simulink model "gm_sampleModel1614_4_sub"  (R2023a)
settings: Solver=VariableStepAuto  StartTime=0.0  StopTime=10.0  RelTol=1e-3
libraries: hdlsllib x1
settings Model: Creator=user1  LastModifiedBy=user1
settings OptimizationCC: BlockReduction=off  ConditionallyExecuteInputs=off
settings DebuggingCC: InheritedTsInSrcMsg=none

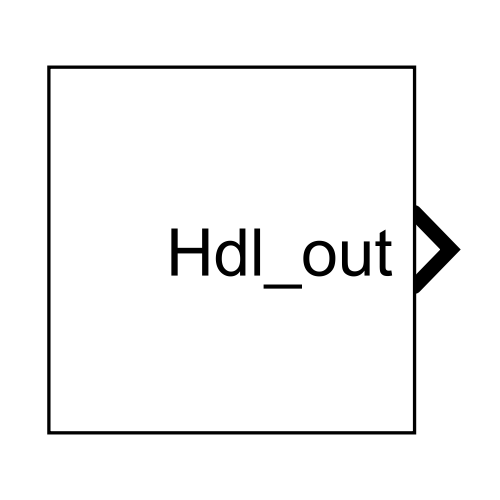
[thumbnail: Simulink's stored preview of the top-level diagram]
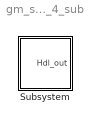
== system gm_sampleModel1614_4_sub ==
  Subsystem : Subsystem

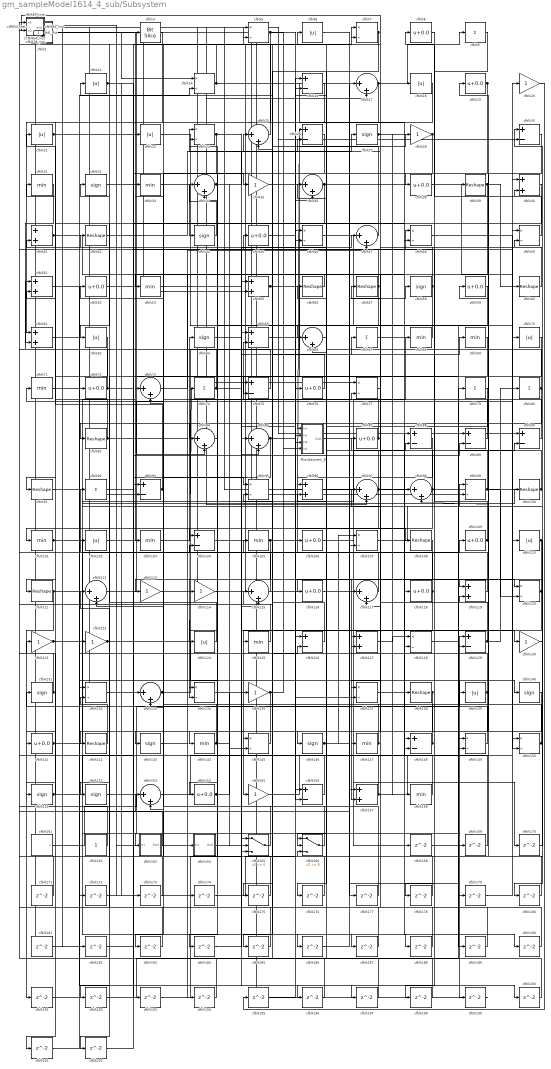
== system gm_sampleModel1614_4_sub/Subsystem ==
  Mysubsystem_8 : Subsystem
  cfblk1 : Subsystem  mask(Detect Rise Nonnegative){vinit=double(0), InputProcessing=Elements as channels (sample based), OutDataTypeStr=uint8}
      mask prompts: vinit "Simulink:masks:InitialCondition_MP"; InputProcessing "Simulink:masks:InputProcessing_MP"; OutDataTypeStr "Simulink:masks:OutputDataType_MP"
      mask help: Simulink:masks:DetectRiseNonnegative_MD
      mask init:
      | InputProcessing = 'Elements as channels (sample based)';
      | OutDataTypeStr = 'uint8';
      | vinit = double(0);
      mask TypeOptions InputProcessing: Simulink:masks:ColumnsAsChannelsFrameBased | Simulink:masks:ElementsAsChannelsSampleBased
      mask TypeOptions OutDataTypeStr: Simulink:masks:uint8 | Simulink:masks:boolean
      mask Display: fprintf('U >= 0\n&  NOT\nU/z >= 0')
  cfblk{39,42,56..57,60,82,91,100,108,111,138,142} (12 alike) : Reshape
  cfblk{31,33,53,68..69,71,101,103,105,125,144,147,158} (13 alike) : MinMax  OutDataTypeStr=uint8
  cfblk{6,12,18,21,23,62,70,102,110,124,139} (11 alike) : Abs  OutDataTypeStr=uint8  SaturateOnIntegerOverflow=off
  cfblk{16,26,30,75,88..90,93,104,126,129,148,156} (13 alike) : Sum  Inputs=+-  OutDataTypeStr=uint8
  cfblk{8,19,38,45,52,59,72,76,87,106,109,116,118,141,154} (15 alike) : Bias  Bias=0.0  SaturateOnIntegerOverflow=off
  cfblk{5,7,14,24,46,48,50,77,95,99,107,120,128,132,134,137,145,149..150} (19 alike) : Product  Inputs=*/  OutDataTypeStr=uint8  RndMeth=Zero  SaturateOnIntegerOverflow=on
  cfblk{17,25,34,36,47,66,73,84..85,97..98,112,115,117,133,153} (16 alike) : Sum  Inputs=|++  OutDataTypeStr=uint8
  cfblk{20,28,35,113..114,121..122,130,135,155} (10 alike) : Gain  OutDataTypeStr=uint8
  cfblk{40..41,51,55,61,65,96,119,127,157} (10 alike) : Sum  OutDataTypeStr=uint8
  cfblk11_inst : Subsystem
  cfblk123_inst : Subsystem
  cfblk{27,32,44,58,64,131,140,143,146,151..152} (11 alike) : Signum
  cfblk136_inst : Subsystem
  cfblk13_inst : Subsystem
  cfblk15_inst : Subsystem
  cfblk161 : Subsystem  mask(Counter Free-Running){NumBits=double(16), tsamp=double(-1)}
      mask prompts: NumBits "Simulink:masks:NumberOfBits_MP"; tsamp "Simulink:masks:SampleTime_MP"
      mask help: Simulink:masks:CounterFreeRunning_MD
  cfblk162 : Constant  OutDataTypeStr=uint8  SampleTime=-1
  cfblk163 : Subsystem
  cfblk164 : Subsystem
  cfblk165 : Switch  OutDataTypeStr=uint8  SaturateOnIntegerOverflow=off  InputSameDT=off
  cfblk166 : Switch  OutDataTypeStr=uint8  SaturateOnIntegerOverflow=off  InputSameDT=off
  cfblk{168..202} (35 alike) : Delay  SampleTime=1
  cfblk2 : Constant  Value=0  OutDataTypeStr=uint8  SampleTime=1
  cfblk22_inst : Subsystem
  cfblk29_inst : Subsystem
  cfblk3 : hdlsllib/Logic and Bit Operations/Bit Slice  lidx=7  ridx=0
  cfblk37_inst : Subsystem
  cfblk43_inst : Subsystem
  cfblk49_inst : Subsystem
  cfblk4_inst : Subsystem
  cfblk54_inst : Subsystem
  cfblk{9,67,74,79..80,92} (6 alike) : Sum  Inputs=+  OutDataTypeStr=uint8
  cfblk78_inst : Subsystem
  cfblk83_inst : Subsystem
  cfblk94_inst : Subsystem
  Hdl_out : Outport  OutDataTypeStr=uint8  SampleTime=1
  wires:
  Mysubsystem_8/1(Out1) -> cfblk168/1
  cfblk1/1(Y) -> cfblk84/2, cfblk14/1
  cfblk100/1 -> cfblk43_inst/2(in2), Hdl_out/1
  cfblk101/1 -> cfblk100/1, cfblk188/1
  cfblk102/1 -> cfblk3/1
  cfblk103/1 -> cfblk64/1
  cfblk104/1 -> cfblk6/1
  cfblk105/1 -> cfblk26/1, cfblk134/2
  cfblk106/1 -> cfblk120/1
  cfblk107/1 -> cfblk50/2
  cfblk108/1 -> cfblk153/2
  cfblk109/1 -> cfblk98/2, cfblk45/1
  cfblk11_inst/1(out1) -> cfblk17/2, cfblk133/1
  cfblk110/1 -> cfblk166/3, cfblk157/2, cfblk180/1
  cfblk111/1 -> cfblk73/1, cfblk109/1, cfblk191/1, cfblk187/1
  cfblk112/1 -> cfblk40/1
  cfblk113/1 -> cfblk28/1
  cfblk114/1 -> cfblk48/1
  cfblk115/1 -> cfblk123_inst/1(in1)
  cfblk116/1 -> cfblk170/1
  cfblk117/1 -> cfblk92/1
  cfblk118/1 -> cfblk25/2, cfblk127/2
  cfblk119/1 -> cfblk15_inst/1(in1)
  cfblk12/1 -> cfblk93/1, cfblk173/1
  cfblk120/1 -> cfblk155/1, cfblk113/1, cfblk125/1
  cfblk121/1 -> cfblk88/2, cfblk99/1
  cfblk122/1 -> cfblk199/1, cfblk74/1
  cfblk123_inst/1(out1) -> cfblk98/1, cfblk164/1(In1)
  cfblk124/1 -> cfblk49_inst/1(in1)
  cfblk125/1 -> cfblk136_inst/1(in1)
  cfblk126/1 -> cfblk5/1
  cfblk127/1 -> cfblk128/1
  cfblk128/1 -> cfblk79/1
  cfblk129/1 -> cfblk15_inst/2(in2), cfblk80/1
  cfblk13_inst/1(out1) -> cfblk99/2, cfblk77/1
  cfblk130/1 -> cfblk40/2
  cfblk131/1 -> cfblk54_inst/2(in2), cfblk201/1
  cfblk132/1 -> cfblk126/2
  cfblk133/1 -> cfblk65/2, cfblk200/1
  cfblk134/1 -> cfblk55/1
  cfblk135/1 -> cfblk183/1, Mysubsystem_8/4(In4)
  cfblk136_inst/1(out1) -> cfblk182/1, cfblk181/1
  cfblk137/1 -> cfblk88/1
  cfblk138/1 -> cfblk192/1, cfblk185/1, cfblk144/1
  cfblk139/1 -> cfblk19/1, cfblk202/1, cfblk105/1
  cfblk14/1 -> cfblk94_inst/1(in1), cfblk148/1
  cfblk140/1 -> cfblk146/1
  cfblk141/1 -> cfblk46/2, cfblk163/1(In1), cfblk68/1
  cfblk142/1 -> cfblk132/2
  cfblk143/1 -> cfblk186/1
  cfblk144/1 -> cfblk52/1, cfblk165/2, cfblk71/1
  cfblk145/1 -> cfblk142/1
  cfblk146/1 -> cfblk177/1, cfblk107/1
  cfblk147/1 -> cfblk29_inst/1(in1), cfblk24/1
  cfblk148/1 -> cfblk66/2, cfblk36/1
  cfblk149/1 -> cfblk131/1
  cfblk15_inst/1(out1) -> cfblk97/2
  cfblk150/1 -> cfblk59/1, cfblk7/1
  cfblk151/1 -> cfblk121/1, cfblk103/1
  cfblk152/1 -> cfblk169/1
  cfblk153/1 -> cfblk89/1
  cfblk154/1 -> cfblk104/2, cfblk135/1
  cfblk155/1 -> cfblk138/1
  cfblk156/1 -> cfblk115/1
  cfblk157/1 -> cfblk87/1, cfblk106/1, cfblk20/1
  cfblk158/1 -> cfblk65/1
  cfblk16/1 -> cfblk141/1
  cfblk161/1(y) -> cfblk129/1
  cfblk162/1 -> cfblk4_inst/1(in1)
  cfblk163/1(Out1) -> cfblk13_inst/2(in2)
  cfblk164/1(Out1) -> cfblk67/1
  cfblk165/1 -> cfblk112/2
  cfblk166/1 -> cfblk22_inst/2(in2)
  cfblk168/1 -> cfblk90/2
  cfblk169/1 -> cfblk123_inst/2(in2)
  cfblk17/1 -> cfblk75/2, cfblk9/1
  cfblk170/1 -> cfblk30/1
  cfblk171/1 -> cfblk94_inst/2(in2)
  cfblk172/1 -> cfblk89/2
  cfblk173/1 -> cfblk29_inst/2(in2)
  cfblk174/1 -> cfblk16/2
  cfblk175/1 -> cfblk153/1
  cfblk176/1 -> cfblk34/2
  cfblk177/1 -> cfblk5/2
  cfblk178/1 -> cfblk97/1
  cfblk179/1 -> cfblk150/1
  cfblk18/1 -> cfblk175/1
  cfblk180/1 -> cfblk119/2
  cfblk181/1 -> cfblk126/1
  cfblk182/1 -> cfblk7/2
  cfblk183/1 -> cfblk49_inst/2(in2)
  cfblk184/1 -> cfblk77/2
  cfblk185/1 -> cfblk132/1
  cfblk186/1 -> cfblk17/1
  cfblk187/1 -> cfblk112/1
  cfblk188/1 -> cfblk117/2
  cfblk189/1 -> cfblk13_inst/1(in1)
  cfblk19/1 -> cfblk75/1, Mysubsystem_8/1(In1)
  cfblk190/1 -> cfblk165/1
  cfblk191/1 -> cfblk157/1
  cfblk192/1 -> cfblk149/2
  cfblk193/1 -> cfblk115/2
  cfblk194/1 -> cfblk11_inst/2(in2)
  cfblk195/1 -> cfblk156/1
  cfblk196/1 -> cfblk54_inst/1(in1)
  cfblk197/1 -> cfblk37_inst/2(in2)
  cfblk198/1 -> cfblk95/2
  cfblk199/1 -> cfblk1/1(U)
  cfblk2/1 -> cfblk174/1
  cfblk20/1 -> cfblk195/1
  cfblk200/1 -> cfblk96/2
  cfblk201/1 -> cfblk14/2
  cfblk202/1 -> cfblk23/1
  cfblk21/1 -> cfblk48/2, cfblk35/1
  cfblk22_inst/1(out1) -> cfblk18/1
  cfblk23/1 -> cfblk139/1
  cfblk24/1 -> cfblk85/1, cfblk133/2
  cfblk25/1 -> cfblk43_inst/1(in1)
  cfblk26/1 -> cfblk156/2
  cfblk27/1 -> cfblk190/1, cfblk158/1
  cfblk28/1 -> cfblk154/1, cfblk184/1
  cfblk29_inst/1(out1) -> cfblk117/1
  cfblk3/1 -> cfblk61/1
  cfblk30/1 -> cfblk149/1
  cfblk31/1 -> cfblk61/2
  cfblk32/1 -> cfblk118/1
  cfblk33/1 -> cfblk44/1
  cfblk34/1 -> cfblk26/2, cfblk145/2, Mysubsystem_8/2(In2)
  cfblk35/1 -> cfblk119/1
  cfblk36/1 -> cfblk62/1, cfblk104/1
  cfblk37_inst/1(out1) -> cfblk30/2
  cfblk38/1 -> cfblk150/2
  cfblk39/1 -> cfblk73/2, cfblk60/1, cfblk127/1
  cfblk4_inst/1(out1) -> cfblk72/1, cfblk122/1
  cfblk40/1 -> cfblk111/1
  cfblk41/1 -> cfblk194/1, cfblk193/1, cfblk128/2
  cfblk42/1 -> cfblk27/1
  cfblk43_inst/1(out1) -> cfblk171/1
  cfblk44/1 -> cfblk34/1
  cfblk45/1 -> cfblk76/1
  cfblk46/1 -> cfblk110/1
  cfblk47/1 -> cfblk12/1
  cfblk48/1 -> cfblk70/1
  cfblk49_inst/1(out1) -> cfblk37_inst/1(in1)
  cfblk5/1 -> cfblk91/1, cfblk36/2, cfblk137/2
  cfblk50/1 -> cfblk8/1
  cfblk51/1 -> cfblk197/1
  cfblk52/1 -> cfblk85/2
  cfblk53/1 -> cfblk46/1
  cfblk54_inst/1(out1) -> cfblk39/1
  cfblk55/1 -> cfblk47/1, cfblk148/2
  cfblk56/1 -> cfblk53/1
  cfblk57/1 -> cfblk83_inst/1(in1), cfblk124/1
  cfblk58/1 -> cfblk24/2, cfblk137/1, Mysubsystem_8/3(In3)
  cfblk59/1 -> cfblk166/2
  cfblk6/1 -> cfblk179/1
  cfblk60/1 -> cfblk11_inst/1(in1)
  cfblk61/1 -> cfblk172/1
  cfblk62/1 -> cfblk151/1
  cfblk64/1 -> cfblk196/1
  cfblk65/1 -> cfblk189/1
  cfblk66/1 -> cfblk96/1
  cfblk67/1 -> cfblk129/2
  cfblk68/1 -> cfblk66/1
  cfblk69/1 -> cfblk198/1
  cfblk7/1 -> cfblk176/1, cfblk145/1
  cfblk70/1 -> cfblk152/1
  cfblk71/1 -> cfblk102/1
  cfblk72/1 -> cfblk78_inst/2(in2), cfblk50/1
  cfblk73/1 -> cfblk47/2
  cfblk74/1 -> cfblk51/2, cfblk51/1, cfblk130/1, cfblk69/1
  cfblk75/1 -> cfblk4_inst/2(in2)
  cfblk76/1 -> cfblk25/1
  cfblk77/1 -> cfblk147/1
  cfblk78_inst/1(out1) -> cfblk93/2, cfblk55/2, cfblk41/1
  cfblk79/1 -> cfblk116/1
  cfblk8/1 -> cfblk178/1
  cfblk80/1 -> cfblk84/1, cfblk82/1, cfblk78_inst/1(in1)
  cfblk82/1 -> cfblk21/1, cfblk114/1
  cfblk83_inst/1(out1) -> cfblk136_inst/2(in2)
  cfblk84/1 -> cfblk134/1
  cfblk85/1 -> cfblk143/1, cfblk107/2
  cfblk87/1 -> cfblk41/2, cfblk22_inst/1(in1)
  cfblk88/1 -> cfblk166/1
  cfblk89/1 -> cfblk57/1
  cfblk9/1 -> cfblk38/1
  cfblk90/1 -> cfblk33/1
  cfblk91/1 -> cfblk140/1
  cfblk92/1 -> cfblk95/1
  cfblk93/1 -> cfblk32/1, cfblk31/1
  cfblk94_inst/1(out1) -> cfblk90/1
  cfblk95/1 -> cfblk108/1
  cfblk96/1 -> cfblk58/1
  cfblk97/1 -> cfblk165/3, cfblk16/1
  cfblk98/1 -> cfblk42/1, cfblk101/1
  cfblk99/1 -> cfblk83_inst/2(in2), cfblk56/1, cfblk120/2

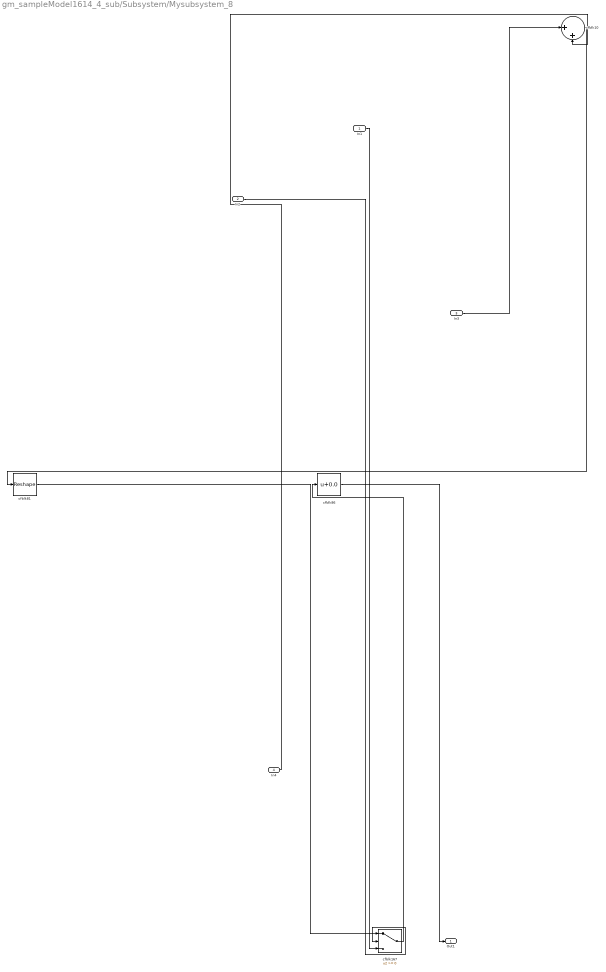
== system gm_sampleModel1614_4_sub/Subsystem/Mysubsystem_8 ==
  In1 : Inport  OutDataTypeStr=uint8  PortDimensions=1  SampleTime=1
  In2 : Inport  Port=2  OutDataTypeStr=uint8  PortDimensions=1  SampleTime=1
  In3 : Inport  Port=3  OutDataTypeStr=uint8  PortDimensions=1  SampleTime=1
  In4 : Inport  Port=4  OutDataTypeStr=uint8  PortDimensions=1  SampleTime=1
  cfblk10 : Sum  Inputs=|++
  cfblk167 : Switch  SaturateOnIntegerOverflow=off  InputSameDT=off
  cfblk81 : Reshape
  cfblk86 : Bias  Bias=0.0  SaturateOnIntegerOverflow=off
  Out1 : Outport  SampleTime=1
  wires:
  In1/1 -> cfblk167/3
  In2/1 -> cfblk167/2
  In3/1 -> cfblk10/1
  In4/1 -> cfblk10/2
  cfblk10/1 -> cfblk81/1
  cfblk167/1 -> cfblk86/1
  cfblk81/1 -> cfblk167/1
  cfblk86/1 -> Out1/1

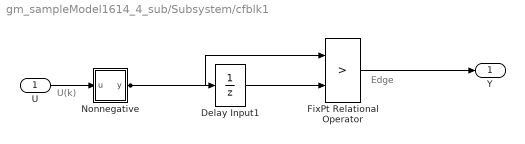
== system gm_sampleModel1614_4_sub/Subsystem/cfblk1 ==
  note: U(k)
  note: Edge
  U : Inport  OutDataTypeStr=uint8  SampleTime=1
  Delay Input1 : UnitDelay  Description=Store in Global RAM  DisableCoverage=on  InitialCondition=vinit  SampleTime=-1  HasFrameUpgradeWarning=on
  FixPt Relational Operator : RelationalOperator  Operator=>  OutDataTypeStr=fixdt(0, 8)  ZeroCross=off  InputSameDT=off
  Nonnegative : Subsystem  mask(Compare To Zero){relop=>=, OutDataTypeStr=boolean, ZeroCross=off}
      mask prompts: relop "Simulink:masks:Operator_MP"; OutDataTypeStr "Simulink:masks:OutputDataType_MP"; ZeroCross "Simulink:masks:EnableZerocrossingDetection_MP"
      mask help: Simulink:masks:CompareToZero_MD
      mask init:
      | OutDataTypeStr = 'boolean';
      | ZeroCross = 'off';
      | blkName = 'sampleModel1614_4_sub/Subsystem/cfblk1/Nonnegative';
      | relop = '>=';
      | setValue = 'boolean';
      mask TypeOptions relop: == | ~= | < | <= | >= | >
      mask TypeOptions OutDataTypeStr: Simulink:masks:uint8 | Simulink:masks:boolean
      mask Callback ZeroCross: sl('zeroCrossEnable', gcbh);
      mask Display: disp([relop,' 0'])
  Y : Outport  SampleTime=1
  wires:
  U/1 -> Nonnegative/1(u)
  Delay Input1/1 -> FixPt Relational Operator/2
  FixPt Relational Operator/1 -> Y/1
  Nonnegative/1(y) -> FixPt Relational Operator/1, Delay Input1/1

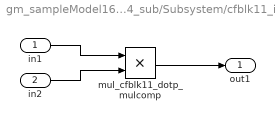
== system gm_sampleModel1614_4_sub/Subsystem/cfblk11_inst ==
  in1 : Inport  OutDataTypeStr=uint8  SampleTime=1
  in2 : Inport  Port=2  OutDataTypeStr=uint8  SampleTime=1
  mul_cfblk11_dotp_mulcomp : Product  Inputs=**  OutDataTypeStr=uint8  SampleTime=1
  out1 : Outport  OutDataTypeStr=uint8  SampleTime=1
  wires:
  in1/1 -> mul_cfblk11_dotp_mulcomp/1
  in2/1 -> mul_cfblk11_dotp_mulcomp/2
  mul_cfblk11_dotp_mulcomp/1 -> out1/1

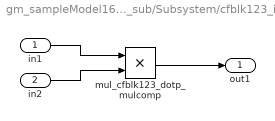
== system gm_sampleModel1614_4_sub/Subsystem/cfblk123_inst ==
  in1 : Inport  OutDataTypeStr=uint8  SampleTime=1
  in2 : Inport  Port=2  OutDataTypeStr=uint8  SampleTime=1
  mul_cfblk123_dotp_mulcomp : Product  Inputs=**  OutDataTypeStr=uint8  SampleTime=1
  out1 : Outport  OutDataTypeStr=uint8  SampleTime=1
  wires:
  in1/1 -> mul_cfblk123_dotp_mulcomp/1
  in2/1 -> mul_cfblk123_dotp_mulcomp/2
  mul_cfblk123_dotp_mulcomp/1 -> out1/1

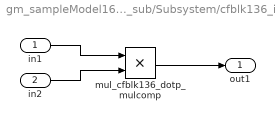
== system gm_sampleModel1614_4_sub/Subsystem/cfblk136_inst ==
  in1 : Inport  OutDataTypeStr=uint8  SampleTime=1
  in2 : Inport  Port=2  OutDataTypeStr=uint8  SampleTime=1
  mul_cfblk136_dotp_mulcomp : Product  Inputs=**  OutDataTypeStr=uint8  SampleTime=1
  out1 : Outport  OutDataTypeStr=uint8  SampleTime=1
  wires:
  in1/1 -> mul_cfblk136_dotp_mulcomp/1
  in2/1 -> mul_cfblk136_dotp_mulcomp/2
  mul_cfblk136_dotp_mulcomp/1 -> out1/1

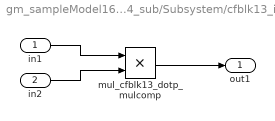
== system gm_sampleModel1614_4_sub/Subsystem/cfblk13_inst ==
  in1 : Inport  OutDataTypeStr=uint8  SampleTime=1
  in2 : Inport  Port=2  OutDataTypeStr=uint8  SampleTime=1
  mul_cfblk13_dotp_mulcomp : Product  Inputs=**  OutDataTypeStr=uint8  SampleTime=1
  out1 : Outport  OutDataTypeStr=uint8  SampleTime=1
  wires:
  in1/1 -> mul_cfblk13_dotp_mulcomp/1
  in2/1 -> mul_cfblk13_dotp_mulcomp/2
  mul_cfblk13_dotp_mulcomp/1 -> out1/1

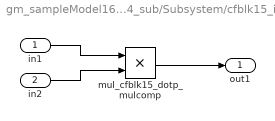
== system gm_sampleModel1614_4_sub/Subsystem/cfblk15_inst ==
  in1 : Inport  OutDataTypeStr=uint8  SampleTime=1
  in2 : Inport  Port=2  OutDataTypeStr=uint8  SampleTime=1
  mul_cfblk15_dotp_mulcomp : Product  Inputs=**  OutDataTypeStr=uint8  SampleTime=1
  out1 : Outport  OutDataTypeStr=uint8  SampleTime=1
  wires:
  in1/1 -> mul_cfblk15_dotp_mulcomp/1
  in2/1 -> mul_cfblk15_dotp_mulcomp/2
  mul_cfblk15_dotp_mulcomp/1 -> out1/1

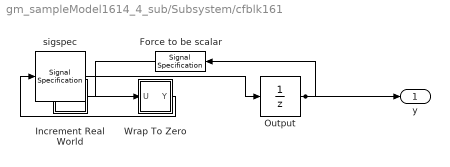
== system gm_sampleModel1614_4_sub/Subsystem/cfblk161 ==
  Force to be scalar : SignalSpecification  DisableCoverage=on  Dimensions=1
  Increment Real World : Subsystem  mask(Real World Value Increment){}
      mask help: Simulink:masks:RealWorldValueIncrement_MD
      mask Display: disp('V++')
  Output : UnitDelay  InitialCondition=0.0  SampleTime=tsamp  HasFrameUpgradeWarning=on
  Wrap To Zero : Subsystem  mask(Wrap To Zero){Threshold=double(65535)}
      mask prompts: Threshold "Simulink:masks:Threshold_MP"
      mask help: Simulink:masks:WrapToZero_MD
  sigspec : SignalSpecification  OutDataTypeStr=uint16  Dimensions=1
  y : Outport  SampleTime=1
  wires:
  Force to be scalar/1 -> Increment Real World/1(u)
  Increment Real World/1(y) -> Wrap To Zero/1(U)
  Output/1 -> Force to be scalar/1, y/1
  Wrap To Zero/1(Y) -> sigspec/1
  sigspec/1 -> Output/1

== system gm_sampleModel1614_4_sub/Subsystem/cfblk163 ==
  In1 : Inport  OutDataTypeStr=uint8  PortDimensions=1  SampleTime=1
  Out1 : Outport  SampleTime=1
  wires:
  In1/1 -> Out1/1

== system gm_sampleModel1614_4_sub/Subsystem/cfblk164 ==
  In1 : Inport  OutDataTypeStr=uint8  PortDimensions=1  SampleTime=1
  Out1 : Outport  SampleTime=1
  wires:
  In1/1 -> Out1/1

== system gm_sampleModel1614_4_sub/Subsystem/cfblk22_inst ==
  in1 : Inport  OutDataTypeStr=uint8  SampleTime=1
  in2 : Inport  Port=2  OutDataTypeStr=uint8  SampleTime=1
  mul_cfblk22_dotp_mulcomp : Product  Inputs=**  OutDataTypeStr=uint8  SampleTime=1
  out1 : Outport  OutDataTypeStr=uint8  SampleTime=1
  wires:
  in1/1 -> mul_cfblk22_dotp_mulcomp/1
  in2/1 -> mul_cfblk22_dotp_mulcomp/2
  mul_cfblk22_dotp_mulcomp/1 -> out1/1

== system gm_sampleModel1614_4_sub/Subsystem/cfblk29_inst ==
  in1 : Inport  OutDataTypeStr=uint8  SampleTime=1
  in2 : Inport  Port=2  OutDataTypeStr=uint8  SampleTime=1
  mul_cfblk29_dotp_mulcomp : Product  Inputs=**  OutDataTypeStr=uint8  SampleTime=1
  out1 : Outport  OutDataTypeStr=uint8  SampleTime=1
  wires:
  in1/1 -> mul_cfblk29_dotp_mulcomp/1
  in2/1 -> mul_cfblk29_dotp_mulcomp/2
  mul_cfblk29_dotp_mulcomp/1 -> out1/1

== system gm_sampleModel1614_4_sub/Subsystem/cfblk37_inst ==
  in1 : Inport  OutDataTypeStr=uint8  SampleTime=1
  in2 : Inport  Port=2  OutDataTypeStr=uint8  SampleTime=1
  mul_cfblk37_dotp_mulcomp : Product  Inputs=**  OutDataTypeStr=uint8  SampleTime=1
  out1 : Outport  OutDataTypeStr=uint8  SampleTime=1
  wires:
  in1/1 -> mul_cfblk37_dotp_mulcomp/1
  in2/1 -> mul_cfblk37_dotp_mulcomp/2
  mul_cfblk37_dotp_mulcomp/1 -> out1/1

== system gm_sampleModel1614_4_sub/Subsystem/cfblk43_inst ==
  in1 : Inport  OutDataTypeStr=uint8  SampleTime=1
  in2 : Inport  Port=2  OutDataTypeStr=uint8  SampleTime=1
  mul_cfblk43_dotp_mulcomp : Product  Inputs=**  OutDataTypeStr=uint8  SampleTime=1
  out1 : Outport  OutDataTypeStr=uint8  SampleTime=1
  wires:
  in1/1 -> mul_cfblk43_dotp_mulcomp/1
  in2/1 -> mul_cfblk43_dotp_mulcomp/2
  mul_cfblk43_dotp_mulcomp/1 -> out1/1

== system gm_sampleModel1614_4_sub/Subsystem/cfblk49_inst ==
  in1 : Inport  OutDataTypeStr=uint8  SampleTime=1
  in2 : Inport  Port=2  OutDataTypeStr=uint8  SampleTime=1
  mul_cfblk49_dotp_mulcomp : Product  Inputs=**  OutDataTypeStr=uint8  SampleTime=1
  out1 : Outport  OutDataTypeStr=uint8  SampleTime=1
  wires:
  in1/1 -> mul_cfblk49_dotp_mulcomp/1
  in2/1 -> mul_cfblk49_dotp_mulcomp/2
  mul_cfblk49_dotp_mulcomp/1 -> out1/1

== system gm_sampleModel1614_4_sub/Subsystem/cfblk4_inst ==
  in1 : Inport  OutDataTypeStr=uint8  SampleTime=1
  in2 : Inport  Port=2  OutDataTypeStr=uint8  SampleTime=1
  mul_cfblk4_dotp_mulcomp : Product  Inputs=**  OutDataTypeStr=uint8  SampleTime=1
  out1 : Outport  OutDataTypeStr=uint8  SampleTime=1
  wires:
  in1/1 -> mul_cfblk4_dotp_mulcomp/1
  in2/1 -> mul_cfblk4_dotp_mulcomp/2
  mul_cfblk4_dotp_mulcomp/1 -> out1/1

== system gm_sampleModel1614_4_sub/Subsystem/cfblk54_inst ==
  in1 : Inport  OutDataTypeStr=uint8  SampleTime=1
  in2 : Inport  Port=2  OutDataTypeStr=uint8  SampleTime=1
  mul_cfblk54_dotp_mulcomp : Product  Inputs=**  OutDataTypeStr=uint8  SampleTime=1
  out1 : Outport  OutDataTypeStr=uint8  SampleTime=1
  wires:
  in1/1 -> mul_cfblk54_dotp_mulcomp/1
  in2/1 -> mul_cfblk54_dotp_mulcomp/2
  mul_cfblk54_dotp_mulcomp/1 -> out1/1

== system gm_sampleModel1614_4_sub/Subsystem/cfblk78_inst ==
  in1 : Inport  OutDataTypeStr=uint8  SampleTime=1
  in2 : Inport  Port=2  OutDataTypeStr=uint8  SampleTime=1
  mul_cfblk78_dotp_mulcomp : Product  Inputs=**  OutDataTypeStr=uint8  SampleTime=1
  out1 : Outport  OutDataTypeStr=uint8  SampleTime=1
  wires:
  in1/1 -> mul_cfblk78_dotp_mulcomp/1
  in2/1 -> mul_cfblk78_dotp_mulcomp/2
  mul_cfblk78_dotp_mulcomp/1 -> out1/1

== system gm_sampleModel1614_4_sub/Subsystem/cfblk83_inst ==
  in1 : Inport  OutDataTypeStr=uint8  SampleTime=1
  in2 : Inport  Port=2  OutDataTypeStr=uint8  SampleTime=1
  mul_cfblk83_dotp_mulcomp : Product  Inputs=**  OutDataTypeStr=uint8  SampleTime=1
  out1 : Outport  OutDataTypeStr=uint8  SampleTime=1
  wires:
  in1/1 -> mul_cfblk83_dotp_mulcomp/1
  in2/1 -> mul_cfblk83_dotp_mulcomp/2
  mul_cfblk83_dotp_mulcomp/1 -> out1/1

== system gm_sampleModel1614_4_sub/Subsystem/cfblk94_inst ==
  in1 : Inport  OutDataTypeStr=uint8  SampleTime=1
  in2 : Inport  Port=2  OutDataTypeStr=uint8  SampleTime=1
  mul_cfblk94_dotp_mulcomp : Product  Inputs=**  OutDataTypeStr=uint8  SampleTime=1
  out1 : Outport  OutDataTypeStr=uint8  SampleTime=1
  wires:
  in1/1 -> mul_cfblk94_dotp_mulcomp/1
  in2/1 -> mul_cfblk94_dotp_mulcomp/2
  mul_cfblk94_dotp_mulcomp/1 -> out1/1

== system gm_sampleModel1614_4_sub/Subsystem/cfblk1/Nonnegative ==
  u : Inport  OutDataTypeStr=uint8  SampleTime=1
  Compare : RelationalOperator  OutDataTypeStr=boolean  ZeroCross=off
  Constant : Constant  DisableCoverage=on  Value=0  OutDataTypeStr=Inherit: Inherit via back propagation  SampleTime=-1  PreserveConstantTs=on
  y : Outport  SampleTime=1
  wires:
  u/1 -> Compare/1
  Compare/1 -> y/1
  Constant/1 -> Compare/2

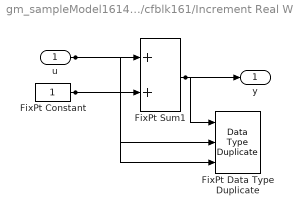
== system gm_sampleModel1614_4_sub/Subsystem/cfblk161/Increment Real World ==
  u : Inport  OutDataTypeStr=uint16  SampleTime=1
  FixPt Constant : Constant  DisableCoverage=on  OutDataTypeStr=Inherit: Inherit via back propagation  SampleTime=-1
  FixPt Data Type Duplicate : DataTypeDuplicate  DisableCoverage=on  NumInputPorts=3
  FixPt Sum1 : Sum  InputSameDT=on  OutDataTypeStr=Inherit: Inherit via back propagation  LockScale=on
  y : Outport  SampleTime=1
  wires:
  u/1 -> FixPt Sum1/1, FixPt Data Type Duplicate/2
  FixPt Constant/1 -> FixPt Sum1/2, FixPt Data Type Duplicate/3
  FixPt Sum1/1 -> FixPt Data Type Duplicate/1, y/1

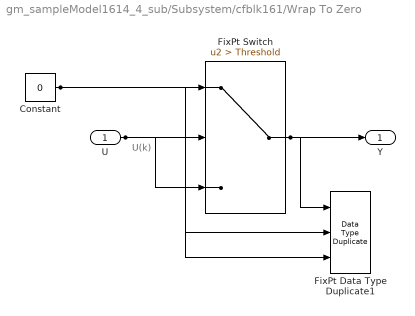
== system gm_sampleModel1614_4_sub/Subsystem/cfblk161/Wrap To Zero ==
  note: U(k)
  U : Inport  OutDataTypeStr=uint16  SampleTime=1
  Constant : Constant  DisableCoverage=on  Value=0  OutDataTypeStr=Inherit: Inherit via back propagation  SampleTime=-1
  FixPt Data Type Duplicate1 : DataTypeDuplicate  DisableCoverage=on  NumInputPorts=3
  FixPt Switch : Switch  Criteria=u2 > Threshold  Threshold=Threshold  OutDataTypeStr=Inherit: Inherit via back propagation  ZeroCross=off  SaturateOnIntegerOverflow=off  InputSameDT=off
  Y : Outport  SampleTime=1
  wires:
  U/1 -> FixPt Switch/3, FixPt Switch/2, FixPt Data Type Duplicate1/2
  Constant/1 -> FixPt Switch/1, FixPt Data Type Duplicate1/3
  FixPt Switch/1 -> FixPt Data Type Duplicate1/1, Y/1
